simulink model "controller_Harness_Warning"  (R2023b)
settings: Solver=FixedStepAuto  StartTime=0.0  StopTime=40  FixedStep=1/100  RelTol=1e-3
libraries: simulink x4
settings Model: Creator=Matteo  LastModifiedBy=dadog
settings OptimizationCC: ReuseModelBlockBuffer=off
settings DebuggingCC: UnconnectedInputMsg=warning  UnconnectedOutputMsg=warning  UnconnectedLineMsg=warning
settings ModelReferenceCC: EnableRefExpFcnMdlSchedulingChecks=on
settings RTWCC: DLArmComputeVersion=19.05
settings ConfigComp: CovEnable=on  CovScope=Subsystem  RecordCoverage=on

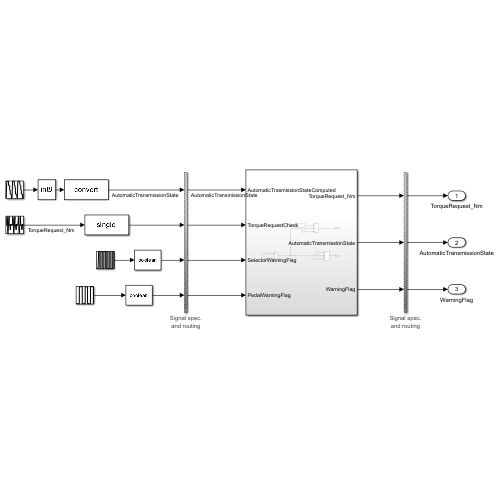
[thumbnail: Simulink's stored preview of the top-level diagram]
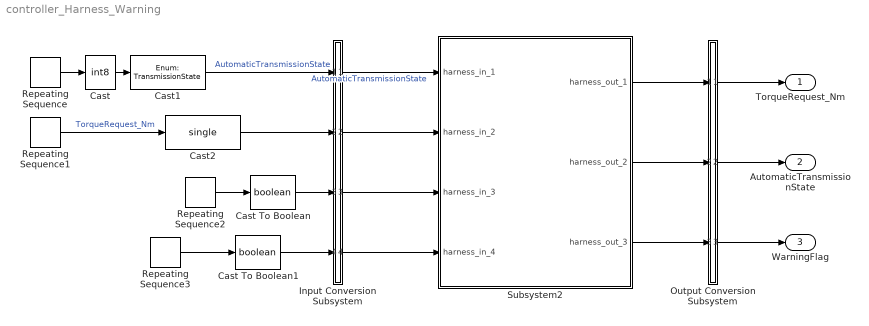
== system controller_Harness_Warning ==
  Cast : DataTypeConversion  OutDataTypeStr=int8  SaturateOnIntegerOverflow=off  RndMeth=Floor
  Cast To Boolean : DataTypeConversion  OutDataTypeStr=boolean  SaturateOnIntegerOverflow=off  RndMeth=Floor
  Cast To Boolean1 : DataTypeConversion  OutDataTypeStr=boolean  SaturateOnIntegerOverflow=off  RndMeth=Floor
  Cast1 : DataTypeConversion  OutDataTypeStr=Enum: TransmissionState  SaturateOnIntegerOverflow=off  RndMeth=Floor
  Cast2 : DataTypeConversion  OutDataTypeStr=single  SaturateOnIntegerOverflow=off  RndMeth=Floor
  Input Conversion Subsystem : Subsystem  Tag=__SLT_ICS__  Description=|
      | Signal spec.
      | and routing
      settings: AttributesFormatString=%<Description>
  Output Conversion Subsystem : Subsystem  Tag=__SLT_OCS__  Description=|
      | Signal spec.
      | and routing
      settings: AttributesFormatString=%<Description>
  Repeating Sequence : simulink/Sources/Repeating Sequence  rep_seq_t=[0 4 17 18 24 25 27.5 28 36 37 40]  rep_seq_y=[0 4 4 3 3 2 2 1 1 0 0]
  Repeating Sequence1 : simulink/Sources/Repeating Sequence  rep_seq_t=[0 4 6 7 8 12 13 14 17 18 20 22 23 24 25 26 27 28 30 35 36 37 38 39 40]  rep_seq_y=[0 0 80 90 80 -80 -90 -80 0 0 90 0 -10 0 0 4 -4 0 -50 10 0 0 5 -5 0]
  Repeating Sequence2 : simulink/Sources/Repeating Sequence  rep_seq_t=[0 10 11 20 21 30 31 40]  rep_seq_y=[0 0 1 1 0 0 1 1]
  Repeating Sequence3 : simulink/Sources/Repeating Sequence  rep_seq_t=[0 10 11 20 21 30 31 40]  rep_seq_y=[0 0 0 0 1 1 1 1]
  Subsystem2 : Subsystem  Tag=__SL_testing_harness_stub_
  TorqueRequest_Nm : Outport
  AutomaticTransmissionState : Outport  Port=2
  WarningFlag : Outport  Port=3
  wires:
  Cast1/1 -> Input Conversion Subsystem/1(Inport_1)  "AutomaticTransmissionState"
  Repeating Sequence2/1 -> Cast To Boolean/1
  Repeating Sequence3/1 -> Cast To Boolean1/1
  Output Conversion Subsystem/1(Outport_1) -> TorqueRequest_Nm/1
  Output Conversion Subsystem/2(Outport_2) -> AutomaticTransmissionState/1
  Output Conversion Subsystem/3(Outport_3) -> WarningFlag/1
  Input Conversion Subsystem/1(Outport_1) -> Subsystem2/1(harness_in_1)  "AutomaticTransmissionState"
  Input Conversion Subsystem/2(Outport_2) -> Subsystem2/2(harness_in_2)
  Input Conversion Subsystem/3(Outport_3) -> Subsystem2/3(harness_in_3)
  Input Conversion Subsystem/4(Outport_4) -> Subsystem2/4(harness_in_4)
  Subsystem2/1(harness_out_1) -> Output Conversion Subsystem/1(Inport_1)
  Subsystem2/2(harness_out_2) -> Output Conversion Subsystem/2(Inport_2)
  Subsystem2/3(harness_out_3) -> Output Conversion Subsystem/3(Inport_3)
  Repeating Sequence/1 -> Cast/1
  Cast/1 -> Cast1/1
  Repeating Sequence1/1 -> Cast2/1  "TorqueRequest_Nm"
  Cast2/1 -> Input Conversion Subsystem/2(Inport_2)
  Cast To Boolean/1 -> Input Conversion Subsystem/3(Inport_3)
  Cast To Boolean1/1 -> Input Conversion Subsystem/4(Inport_4)

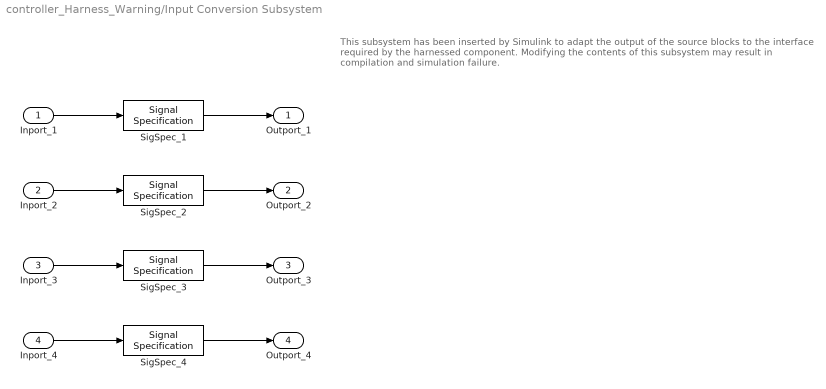
== system controller_Harness_Warning/Input Conversion Subsystem ==
  note: This subsystem has been inserted by Simulink to adapt the output of the source blocks to the interface required by the harnessed component.
      |  Modifying the contents of this subsystem may result in compilation and simulation failure.
  Inport_1 : Inport
  Inport_2 : Inport  Port=2
  Inport_3 : Inport  Port=3
  Inport_4 : Inport  Port=4
  SigSpec_1 : SignalSpecification  OutDataTypeStr=Enum: TransmissionState  Dimensions=[1]  SampleTime=0.01
  SigSpec_2 : SignalSpecification  OutDataTypeStr=single  Dimensions=[1]  SampleTime=0.01
  SigSpec_3 : SignalSpecification  OutDataTypeStr=boolean  Dimensions=[1]  SampleTime=0.01
  SigSpec_4 : SignalSpecification  OutDataTypeStr=boolean  Dimensions=[1]  SampleTime=0.01
  Outport_1 : Outport
  Outport_2 : Outport  Port=2
  Outport_3 : Outport  Port=3
  Outport_4 : Outport  Port=4
  wires:
  SigSpec_1/1 -> Outport_1/1
  Inport_1/1 -> SigSpec_1/1
  SigSpec_2/1 -> Outport_2/1
  Inport_2/1 -> SigSpec_2/1
  SigSpec_3/1 -> Outport_3/1
  Inport_3/1 -> SigSpec_3/1
  SigSpec_4/1 -> Outport_4/1
  Inport_4/1 -> SigSpec_4/1

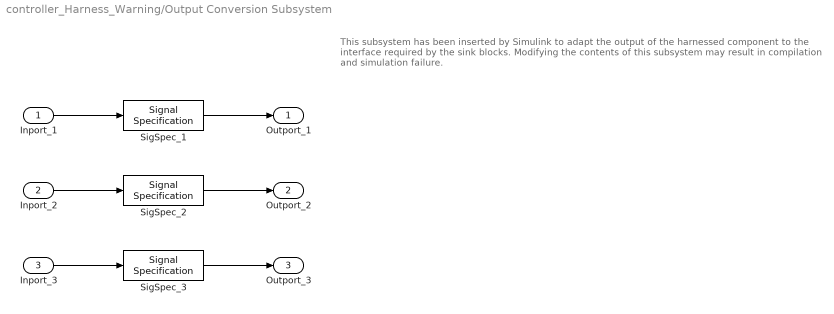
== system controller_Harness_Warning/Output Conversion Subsystem ==
  note: This subsystem has been inserted by Simulink to adapt the output of the harnessed component to the interface required by the sink blocks.
      |  Modifying the contents of this subsystem may result in compilation and simulation failure.
  Inport_1 : Inport
  Inport_2 : Inport  Port=2
  Inport_3 : Inport  Port=3
  SigSpec_1 : SignalSpecification  OutDataTypeStr=single  Unit=N*m  Dimensions=[1]  SampleTime=0.01
  SigSpec_2 : SignalSpecification  OutDataTypeStr=Enum: TransmissionState  Dimensions=[1]  SampleTime=0.01
  SigSpec_3 : SignalSpecification  OutDataTypeStr=boolean  Dimensions=[1]  SampleTime=0.01
  Outport_1 : Outport
  Outport_2 : Outport  Port=2
  Outport_3 : Outport  Port=3
  wires:
  Inport_1/1 -> SigSpec_1/1
  SigSpec_1/1 -> Outport_1/1
  Inport_2/1 -> SigSpec_2/1
  SigSpec_2/1 -> Outport_2/1
  Inport_3/1 -> SigSpec_3/1
  SigSpec_3/1 -> Outport_3/1

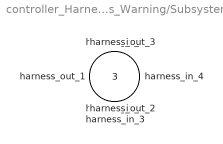
== system controller_Harness_Warning/Subsystem2 ==
  harness_in_1 : Inport
  harness_in_2 : Inport  Port=2
  harness_in_3 : Inport  Port=3
  harness_in_4 : Inport  Port=4
  harness_out_1 : Outport
  harness_out_2 : Outport  Port=2
  harness_out_3 : Outport  Port=3
